simulink model "b_r309c_med"  (Simulink 6.2)
settings: Solver=ode45  StartTime=0.0  StopTime=1030.0  RelTol=1e-3
undefined symbols (not defined in the file): ant_bits, BEE2_usr, blockCountBits, blockRowBits, cmult_4bit_em
libraries: xbsIndex_r3 x2808, xps_library x97, casper_library x84
(part 1 of 20)
settings Model: LastModifiedBy=dsp
settings DebuggingCC: SolverPrmCheckMsg=warning

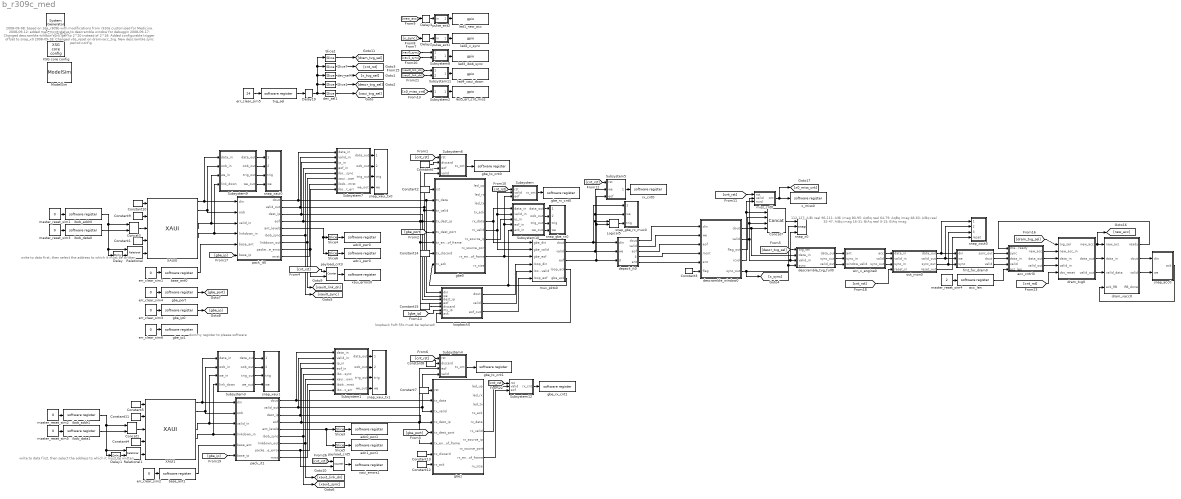
== system b_r309c_med ==
  note: 2008-09-08: based on 16a_r309b with modifications from r310a
      | customised for Medicina.
      |
      | 2008-09-12: added max_mcnt status to descramble window for debuggin
      |
      | 2008-09-17:
      | Changed descramble window sync gen to 2^20 instead of 2^18.
      | Added configurable trigger offset to snap_x0
      |
      | 2008-09-18:
      | Changed vbs_reset on dramvacc_tvg.
      | New descramble sync period config
  note: 112-127: AiBi real
      | 96-111: AiBi imag
      | 80-95: AqBq real
      | 64-79: AqBq imag
      | 48-63: AiBq real
      | 32-47: AiBq imag
      | 16-31: BiAq real
      | 0-15: BiAq imag
  note: write to data first,
      | then select the address
      | to which it must be written
  note: write to data first,
      | then select the address
      | to which it must be written
  note: loopback fwft fifo must be replaced!
  note: dummy register
      | to please software
  " System Generator" : xbsIndex_r3/ System Generator  Tag=genX  xilinxfamily=Virtex2P  part=xc2vp70  speed=-7  package=ff1704  synthesis_tool=XST  directory=./b_r309c_med/sysgen  testbench=off  simulink_period=1  sysclk_period=4.878  incr_netlist=off  trim_vbits=Everywhere in SubSystem  dbl_ovrd=According to Block Masks  core_generation=According to Block Masks  run_coregen=off  deprecated_control=off  eval_field=0
      settings: AttributesFormatString=System\nGenerator
  Concat1 : xbsIndex_r3/Concat  num_inputs=2  explicit_period=off  period=1  dbl_ovrd=off
  Concat3 : xbsIndex_r3/Concat  num_inputs=2  explicit_period=off  period=1  dbl_ovrd=off
  Concat7 : xbsIndex_r3/Concat  num_inputs=4  explicit_period=off  period=1  dbl_ovrd=off
  Constant1 : xbsIndex_r3/Constant  const=0  equ=P=C  arith_type=Unsigned  n_bits=64  bin_pt=0  opselect=C  inp2=PCIN>>17  opr=+  inp1=P  carry=CIN  iostate=0  explicit_period=on  period=1  dbl_ovrd=off
  Constant10 : xbsIndex_r3/Constant  const=1  equ=P=C  arith_type=Boolean  n_bits=1  bin_pt=0  opselect=C  inp2=PCIN>>17  opr=+  inp1=P  carry=CIN  iostate=0  explicit_period=on  period=1  dbl_ovrd=off
  Constant{2,6..7,9,11,14..15} (7 alike) : xbsIndex_r3/Constant  const=0  equ=P=C  arith_type=Boolean  n_bits=1  bin_pt=0  opselect=C  inp2=PCIN>>17  opr=+  inp1=P  carry=CIN  iostate=0  explicit_period=on  period=1  dbl_ovrd=off
  Constant12 : xbsIndex_r3/Constant  const=1  equ=P=C  arith_type=Boolean  n_bits=16  bin_pt=0  opselect=C  inp2=PCIN>>17  opr=+  inp1=P  carry=CIN  iostate=0  explicit_period=on  period=1  dbl_ovrd=off
  Constant13 : xbsIndex_r3/Constant  const=0  equ=P=C  arith_type=Boolean  n_bits=16  bin_pt=0  opselect=C  inp2=PCIN>>17  opr=+  inp1=P  carry=CIN  iostate=0  explicit_period=on  period=1  dbl_ovrd=off
  Constant3 : xbsIndex_r3/Constant  const=0  equ=P=C  arith_type=Unsigned  n_bits=1  bin_pt=0  opselect=C  inp2=PCIN>>17  opr=+  inp1=P  carry=CIN  iostate=0  explicit_period=on  period=1  dbl_ovrd=off
  Constant4 : xbsIndex_r3/Constant  const=0  equ=P=C  arith_type=Unsigned  n_bits=64  bin_pt=0  opselect=C  inp2=PCIN>>17  opr=+  inp1=P  carry=CIN  iostate=0  explicit_period=on  period=1  dbl_ovrd=off
  Constant5 : xbsIndex_r3/Constant  const=1  equ=P=C  arith_type=Boolean  n_bits=1  bin_pt=0  opselect=C  inp2=PCIN>>17  opr=+  inp1=P  carry=CIN  iostate=0  explicit_period=on  period=1  dbl_ovrd=off
  Constant8 : xbsIndex_r3/Constant  const=0  equ=P=C  arith_type=Boolean  n_bits=16  bin_pt=0  opselect=C  inp2=PCIN>>17  opr=+  inp1=P  carry=CIN  iostate=0  explicit_period=on  period=1  dbl_ovrd=off
  Delay{,1..3} (4 alike) : xbsIndex_r3/Delay  latency=1  reg_retiming=on  explicit_period=off  period=1  en=off  accept_only_valid=off  init_zero=on  dbl_ovrd=off  show_param=off
      settings: xl_area=[0, 0, 0, 0, 0, 0, 0]
  Delay19 : xbsIndex_r3/Delay  latency=2  reg_retiming=on  explicit_period=off  period=1  en=off  accept_only_valid=off  init_zero=on  dbl_ovrd=off  show_param=off
      settings: xl_area=[0, 0, 0, 0, 0, 0, 0]
  Logical5 : xbsIndex_r3/Logical  logical_function=AND  inputs=2  precision=Full  arith_type=Unsigned  n_bits=8  bin_pt=2  align_bp=on  latency=0  explicit_period=off  period=1  en=off  dbl_ovrd=off  show_param=off
      settings: xl_area=[0, 0, 0, 0, 0, 0, 0]
  ModelSim : xbsIndex_r3/ModelSim  dir=./modelsim  waveform=on  leave_open=on  skip_compile=off  custom_scripts=off  startup_timeout=40
  Relational : xbsIndex_r3/Relational  mode=a!=b  latency=0  explicit_period=off  period=1  en=off  dbl_ovrd=off  show_param=off
      settings: xl_area=[0, 0, 0, 0, 0, 0, 0]
  Relational1 : xbsIndex_r3/Relational  mode=a!=b  latency=0  explicit_period=off  period=1  en=off  dbl_ovrd=off  show_param=off
      settings: xl_area=[0, 0, 0, 0, 0, 0, 0]
  Slice1 : xbsIndex_r3/Slice  mode=Lower Bit Location + Width  nbits=2  bit1=0  base1=MSB of Input  bit0=1  base0=LSB of Input  boolean_output=off  explicit_period=off  period=1  dbl_ovrd=off
  Slice2 : xbsIndex_r3/Slice  mode=Lower Bit Location + Width  nbits=6  bit1=0  base1=MSB of Input  bit0=9  base0=LSB of Input  boolean_output=off  explicit_period=off  period=1  dbl_ovrd=off
  Slice3 : xbsIndex_r3/Slice  mode=Lower Bit Location + Width  nbits=32  bit1=0  base1=MSB of Input  bit0=32  base0=LSB of Input  boolean_output=off  explicit_period=off  period=1  dbl_ovrd=off
  Slice4 : xbsIndex_r3/Slice  mode=Lower Bit Location + Width  nbits=32  bit1=0  base1=MSB of Input  bit0=32  base0=LSB of Input  boolean_output=off  explicit_period=off  period=1  dbl_ovrd=off
  Slice5 : xbsIndex_r3/Slice  mode=Lower Bit Location + Width  nbits=32  bit1=0  base1=MSB of Input  bit0=0  base0=LSB of Input  boolean_output=off  explicit_period=off  period=1  dbl_ovrd=off
  Slice6 : xbsIndex_r3/Slice  mode=Lower Bit Location + Width  nbits=32  bit1=0  base1=MSB of Input  bit0=0  base0=LSB of Input  boolean_output=off  explicit_period=off  period=1  dbl_ovrd=off
  Slice7 : xbsIndex_r3/Slice  mode=Lower Bit Location + Width  nbits=1  bit1=0  base1=MSB of Input  bit0=8  base0=LSB of Input  boolean_output=on  explicit_period=off  period=1  dbl_ovrd=off
  Subsystem : Subsystem
  Subsystem1 : Subsystem
  Subsystem10 : Subsystem
  Subsystem11 : Subsystem
  Subsystem12 : Subsystem
  Subsystem2 : Subsystem
  Subsystem3 : Subsystem
  Subsystem4 : Subsystem
  Subsystem5 : Subsystem
  Subsystem6 : Subsystem
  Subsystem7 : Subsystem
  Subsystem8 : Subsystem
  Subsystem9 : Subsystem
  XAUI0 : xps_library/XAUI  Tag=xps:xaui  demux=1  port=BEE2_usr:0  show_param=off  pre_emph=3  swing=800
  XAUI1 : xps_library/XAUI  Tag=xps:xaui  demux=1  port=BEE2_usr:1  show_param=on  pre_emph=3  swing=800
  XSG core config : xps_library/XSG core config  Tag=xps:xsg  hw_sys=BEE2_usr  ibob_linux=off  clk_src=sys_clk2x  gpio_clk_io_group=iBOB:sma  gpio_clk_bit_index=0  clk_rate=205  sample_period=1  synthesis_tool=XST  mpc_type=powerpc405
  acc_cntrl0 : Subsystem
  acc_len : xps_library/software register  Tag=xps:sw_reg  io_dir=From Processor  arith_type=Unsigned  bitwidth=32  bin_pt=0  sample_period=1  gw_name=b_r309c_med_acc_len_user_data_out
  adc0_pwr0 : xps_library/software register  Tag=xps:sw_reg  io_dir=To Processor  arith_type=Unsigned  bitwidth=32  bin_pt=0  sample_period=1  gw_name=b_r309c_med_adc0_pwr0_user_data_in
  adc0_pwr1 : xps_library/software register  Tag=xps:sw_reg  io_dir=To Processor  arith_type=Unsigned  bitwidth=32  bin_pt=0  sample_period=1  gw_name=b_r309c_med_adc0_pwr1_user_data_in
  adc1_pwr0 : xps_library/software register  Tag=xps:sw_reg  io_dir=To Processor  arith_type=Unsigned  bitwidth=32  bin_pt=0  sample_period=1  gw_name=b_r309c_med_adc1_pwr0_user_data_in
  adc1_pwr1 : xps_library/software register  Tag=xps:sw_reg  io_dir=To Processor  arith_type=Unsigned  bitwidth=32  bin_pt=0  sample_period=1  gw_name=b_r309c_med_adc1_pwr1_user_data_in
  base_ant0 : xps_library/software register  Tag=xps:sw_reg  io_dir=From Processor  arith_type=Unsigned  bitwidth=32  bin_pt=0  sample_period=1  gw_name=b_r309c_med_base_ant0_user_data_out
  base_ant1 : xps_library/software register  Tag=xps:sw_reg  io_dir=From Processor  arith_type=Unsigned  bitwidth=32  bin_pt=0  sample_period=1  gw_name=b_r309c_med_base_ant1_user_data_out
  depack_it0 : Subsystem  mask{payload_len=32}
      mask prompts: payload_len "Payload Length"
      mask init:
      | payload_bits = ceil(log2(payload_len));
      | packet_len = payload_len + 1;
      | packet_bits = ceil(log2(packet_len));
  descramble_tvg_full0 : Subsystem  mask{ant_bits=4, x_int_bits=7, sync_period=20}
      mask prompts: ant_bits "Number of Antennas (2^?):"; x_int_bits "X Integration Length (2^?):"; sync_period "Sync Pulse Period (2^?):"
  descramble_window0 : Subsystem  mask{ant_bits=4, x_int_bits=7, window_bits=3, n_chans=2048, n_xeng=4}
      mask prompts: ant_bits "Maximum Number of Antennas (2^?):"; x_int_bits "X Engine Integration Length (2^?):"; window_bits "Number of Windows to Buffer (2^?):"; n_chans "Number of frequency channels in the system"; n_xeng "Number of Xengines in the system"
      mask init:
      | sync_clks=n_chans/n_xeng*(2^x_int_bits)*(2^ant_bits)
      | 
      | sync_bits=ceil(log2(sync_clks))
      | 
      | fmtstr = sprintf('Sync period: 2^%d', sync_bits);
      | set_param(gcb, 'AttributesFormatString', fmtstr);
      settings: AttributesFormatString=Sync period: 2^20
  dev_sel1 : xbsIndex_r3/Slice  mode=Lower Bit Location + Width  nbits=1  bit1=0  base1=MSB of Input  bit0=0  base0=LSB of Input  boolean_output=off  explicit_period=off  period=1  dbl_ovrd=off
  dev_sel4 : xbsIndex_r3/Slice  mode=Lower Bit Location + Width  nbits=2  bit1=0  base1=MSB of Input  bit0=3  base0=LSB of Input  boolean_output=off  explicit_period=off  period=1  dbl_ovrd=off
  dram_tvg0 : Subsystem  mask{len=(2048/4) * (16*17/2) * 4 * 2 / 4}
      mask prompts: len "Number of Vectors"
      mask init:
      | fmtstr = sprintf('Vector Length: %d', len);
      | set_param(gcb, 'AttributesFormatString', fmtstr);
      settings: AttributesFormatString=Vector Length: 139264
  dram_vacc0 : Subsystem  mask{acc_length=139264}
      mask prompts: acc_length "Vector length??(# cycles)"
      mask init:
      | valid_length = 36;
  err_clear_sim{1..4,6} (5 alike) : Constant  Value=0
  err_clear_sim5 : Constant  Value=24
  fmt_for_dram0 : Subsystem  mask{x_int_bits=7, x_n_bits=4}
      mask prompts: x_int_bits "X Engine integration length (2^?):"; x_n_bits "X Engine input bits"
  gbe0 : Subsystem  Tag=xps:tengbe  AncestorBlock=xps_library/ten_GbE  mask{port=BEE2_usr:2, mac_lite=on, show_param=off, pre_emph=3, swing=800}
      mask prompts: mac_lite "Use light-weight MAC: Warning --> it DOES NOT check any CRC on receive"; show_param "---------------------- Show Implementation Parameters -----------------------------------------------------------------------------------"; pre_emph "Pre-emphasis"; swing "Differential swing"
      mask init:
      | tengbe_mask;
      mask StyleString: popup(iBOB:0|iBOB:1|BEE2_ctrl:0|BEE2_ctrl:1|BEE2_usr:0|BEE2_usr:1|BEE2_usr:2|BEE2_usr:3|CORR:0),checkbox,checkbox,popup(0|1|2|3),popup(400|500|600|700|800)
      mask CallbackString:
      | ||myname=gcb;
      | if strcmp(get_param(myname, 'show_param'), 'on')
      |     set_param(myname, 'MaskVisibilities', {'on','on','on','on', 'on'});
      | else
      |     set_param(myname, 'MaskVisibilities', {'on','on','on','off','off'});
      | end||
  gbe1 : Subsystem  Tag=xps:tengbe  AncestorBlock=xps_library/ten_GbE  mask{port=BEE2_usr:3, mac_lite=on, show_param=off, pre_emph=3, swing=800}
      mask prompts: mac_lite "Use light-weight MAC: Warning --> it DOES NOT check any CRC on receive"; show_param "---------------------- Show Implementation Parameters -----------------------------------------------------------------------------------"; pre_emph "Pre-emphasis"; swing "Differential swing"
      mask init:
      | tengbe_mask;
      mask StyleString: popup(iBOB:0|iBOB:1|BEE2_ctrl:0|BEE2_ctrl:1|BEE2_usr:0|BEE2_usr:1|BEE2_usr:2|BEE2_usr:3|CORR:0),checkbox,checkbox,popup(0|1|2|3),popup(400|500|600|700|800)
      mask CallbackString:
      | ||myname=gcb;
      | if strcmp(get_param(myname, 'show_param'), 'on')
      |     set_param(myname, 'MaskVisibilities', {'on','on','on','on', 'on'});
      | else
      |     set_param(myname, 'MaskVisibilities', {'on','on','on','off','off'});
      | end||
  gbe_ip0 : xps_library/software register  Tag=xps:sw_reg  io_dir=From Processor  arith_type=Unsigned  bitwidth=32  bin_pt=0  sample_period=1  gw_name=b_r309c_med_gbe_ip0_user_data_out
  gbe_ip1 : xps_library/software register  Tag=xps:sw_reg  io_dir=From Processor  arith_type=Unsigned  bitwidth=32  bin_pt=0  sample_period=1  gw_name=b_r309c_med_gbe_ip1_user_data_out
  gbe_port : xps_library/software register  Tag=xps:sw_reg  io_dir=From Processor  arith_type=Unsigned  bitwidth=32  bin_pt=0  sample_period=1  gw_name=b_r309c_med_gbe_port_user_data_out
  gbe_rx_cnt0 : xps_library/software register  Tag=xps:sw_reg  io_dir=To Processor  arith_type=Unsigned  bitwidth=32  bin_pt=0  sample_period=1  gw_name=b_r309c_med_gbe_rx_cnt0_user_data_in
  gbe_rx_cnt1 : xps_library/software register  Tag=xps:sw_reg  io_dir=To Processor  arith_type=Unsigned  bitwidth=32  bin_pt=0  sample_period=1  gw_name=b_r309c_med_gbe_rx_cnt1_user_data_in
  gbe_tx_cnt0 : xps_library/software register  Tag=xps:sw_reg  io_dir=To Processor  arith_type=Unsigned  bitwidth=32  bin_pt=0  sample_period=1  gw_name=b_r309c_med_gbe_tx_cnt0_user_data_in
  gbe_tx_cnt1 : xps_library/software register  Tag=xps:sw_reg  io_dir=To Processor  arith_type=Unsigned  bitwidth=32  bin_pt=0  sample_period=1  gw_name=b_r309c_med_gbe_tx_cnt1_user_data_in
  ibob_addr0 : xps_library/software register  Tag=xps:sw_reg  io_dir=From Processor  arith_type=Unsigned  bitwidth=32  bin_pt=0  sample_period=1  gw_name=b_r309c_med_ibob_addr0_user_data_out
  ibob_addr1 : xps_library/software register  Tag=xps:sw_reg  io_dir=From Processor  arith_type=Unsigned  bitwidth=32  bin_pt=0  sample_period=1  gw_name=b_r309c_med_ibob_addr1_user_data_out
  ibob_data0 : xps_library/software register  Tag=xps:sw_reg  io_dir=From Processor  arith_type=Unsigned  bitwidth=32  bin_pt=0  sample_period=1  gw_name=b_r309c_med_ibob_data0_user_data_out
  ibob_data1 : xps_library/software register  Tag=xps:sw_reg  io_dir=From Processor  arith_type=Unsigned  bitwidth=32  bin_pt=0  sample_period=1  gw_name=b_r309c_med_ibob_data1_user_data_out
  led1_new_acc : xps_library/gpio  Tag=xps:gpio  io_group=BEE2_usr:led  io_dir=out  arith_type=Boolean  bitwidth=1  bin_pt=0  bit_index=0  sample_period=1  use_single_ended=off  use_ddr=off  reg_iob=off  reg_clk_phase=0  termination=None
  led2_x_sync : xps_library/gpio  Tag=xps:gpio  io_group=BEE2_usr:led  io_dir=out  arith_type=Boolean  bitwidth=1  bin_pt=0  bit_index=1  sample_period=1  use_single_ended=off  use_ddr=off  reg_iob=off  reg_clk_phase=0  termination=None
  led3_ibob_sync : xps_library/gpio  Tag=xps:gpio  io_group=BEE2_usr:led  io_dir=out  arith_type=Boolean  bitwidth=1  bin_pt=0  bit_index=2  sample_period=1  use_single_ended=off  use_ddr=off  reg_iob=off  reg_clk_phase=0  termination=None
  led4_xaui_down : xps_library/gpio  Tag=xps:gpio  io_group=BEE2_usr:led  io_dir=out  arith_type=Boolean  bitwidth=1  bin_pt=0  bit_index=3  sample_period=1  use_single_ended=off  use_ddr=off  reg_iob=off  reg_clk_phase=0  termination=None
  led5_err_cnt_miss : xps_library/gpio  Tag=xps:gpio  io_group=BEE2_usr:led  io_dir=out  arith_type=Boolean  bitwidth=1  bin_pt=0  bit_index=4  sample_period=1  use_single_ended=off  use_ddr=off  reg_iob=off  reg_clk_phase=0  termination=None
  loopback0 : Subsystem  mask{depth_bits=8}
      mask prompts: depth_bits "Buffer Size (2^?):"
      mask help: A loopback is a buffer for holding packets which are to be transmitted to one's self. Most switches drop any packets which have a destination IP address equal to the address of the transmitter. Thus, a seperate buffer is needed to collect these packets for readback.
  master_reset_sim{1..3,5} (4 alike) : Constant  Value=0
  master_reset_sim4 : Constant  Value=2
  miss_cnt0 : Subsystem
  mux_pkts0 : Subsystem
  out_mon0 : Subsystem  mask{n_ants=16, n_chans=2048, n_xeng=4}
      mask prompts: n_ants "Number of Antennas"; n_chans "Number of Frequency Channels in the system"; n_xeng "Number of X engines"
  pack_it0 : Subsystem  mask{payload_len=32, ant_bits=4, xeng_bits=2, skip_xeng_bits=0, skip_ant_bits=1}
      mask prompts: payload_len "Payload Length (in 64 bit words)"; ant_bits "Number of Antennas (2^?)"; xeng_bits "Number of X engines (2^?)"; skip_xeng_bits "X engines per IP address (2^?)"; skip_ant_bits "Antennas per XAUI link (2^?)"
      mask help: Packetizes data coming in over a XAUI interface. A packet consists of a 64 bit header (48 bits of "mcnt" and 16 bits of antenna), followed by 64 x "payload" bits of payload. "Mcnt" (master count) is a counter which keeps track of how many packets have been transmitted since the last "mrst".
      mask init:
      | packet_len = payload_len + 1;
      | packet_bits = ceil(log2(packet_len));
      | payload_bits = ceil(log2(payload_len));
  pack_it1 : Subsystem  mask{payload_len=32, ant_bits=4, xeng_bits=2, skip_xeng_bits=0, skip_ant_bits=1}
      mask prompts: payload_len "Payload Length (in 64 bit words)"; ant_bits "Number of Antennas (2^?)"; xeng_bits "Number of X engines (2^?)"; skip_xeng_bits "X engines per IP address (2^?)"; skip_ant_bits "Antennas per XAUI link (2^?)"
      mask help: Packetizes data coming in over a XAUI interface. A packet consists of a 64 bit header (48 bits of "mcnt" and 16 bits of antenna), followed by 64 x "payload" bits of payload. "Mcnt" (master count) is a counter which keeps track of how many packets have been transmitted since the last "mrst".
      mask init:
      | packet_len = payload_len + 1;
      | packet_bits = ceil(log2(packet_len));
      | payload_bits = ceil(log2(payload_len));
  payload_cnt3 : xbsIndex_r3/Counter  cnt_type=Free Running  n_bits=32  bin_pt=0  arith_type=Unsigned  start_count=0  cnt_to=0  cnt_by_val=1  operation=Up  explicit_period=off  period=1  load_pin=off  rst=on  en=on  dbl_ovrd=off  show_param=off  use_rpm=on  gen_core=off
      settings: xl_area=[0, 0, 0, 0, 0, 0, 0]
  payload_cnt5 : xbsIndex_r3/Counter  cnt_type=Free Running  n_bits=32  bin_pt=0  arith_type=Unsigned  start_count=0  cnt_to=0  cnt_by_val=1  operation=Up  explicit_period=off  period=1  load_pin=off  rst=on  en=on  dbl_ovrd=off  show_param=off  use_rpm=on  gen_core=off
      settings: xl_area=[0, 0, 0, 0, 0, 0, 0]
  pulse_ext1 : Subsystem  mask{pulse_len=2^23}
      mask prompts: pulse_len "Length of Pulse"
      mask init:
      | bits = ceil(log2(pulse_len));
  pulse_ext2 : Subsystem  mask{pulse_len=2^23}
      mask prompts: pulse_len "Length of Pulse"
      mask init:
      | bits = ceil(log2(pulse_len));
  rx_cnt0 : xps_library/software register  Tag=xps:sw_reg  io_dir=To Processor  arith_type=Unsigned  bitwidth=32  bin_pt=0  sample_period=1  gw_name=b_r309c_med_rx_cnt0_user_data_in
  snap_acc0 : Subsystem
  snap_gbe_rx0 : Subsystem  AncestorBlock=casper_library/Scopes/snap64  mask(snap64){nsamples=11}
      mask prompts: nsamples "No. of samples(2^?)"
      mask help:
      | The <i>snap</i> block provides a packaged solution to capturing data from
      | the FPGA fabric and making it accessible from the CPU.  The block comes in
      | 2 flavors: <i>snap</i> (which captures to a 32 bit wide Shared BRAM), and
      | <i>snap64</i> (which captures to 2x32 bit wide Shared BRAMs to effect a
      | 64 bit capture).
      mask Help: eval('xlWeb([getenv(''MLIB_ROOT''), ''\casper_library\doc\snap_usage.html''])')
  snap_gbe_rx_mux0 : Subsystem  AncestorBlock=casper_library/Scopes/snap64  mask(snap64){nsamples=12}
      mask prompts: nsamples "No. of samples(2^?)"
      mask help:
      | The <i>snap</i> block provides a packaged solution to capturing data from
      | the FPGA fabric and making it accessible from the CPU.  The block comes in
      | 2 flavors: <i>snap</i> (which captures to a 32 bit wide Shared BRAM), and
      | <i>snap64</i> (which captures to 2x32 bit wide Shared BRAMs to effect a
      | 64 bit capture).
      mask Help: eval('xlWeb([getenv(''MLIB_ROOT''), ''\casper_library\doc\snap_usage.html''])')
  snap_x0 : casper_library/Scopes/snap  nsamples=12
  snap_xaui0 : Subsystem  AncestorBlock=casper_library/Scopes/snap64  mask(snap64){nsamples=12}
      mask prompts: nsamples "No. of samples(2^?)"
      mask help:
      | The <i>snap</i> block provides a packaged solution to capturing data from
      | the FPGA fabric and making it accessible from the CPU.  The block comes in
      | 2 flavors: <i>snap</i> (which captures to a 32 bit wide Shared BRAM), and
      | <i>snap64</i> (which captures to 2x32 bit wide Shared BRAMs to effect a
      | 64 bit capture).
      mask Help: eval('xlWeb([getenv(''MLIB_ROOT''), ''\casper_library\doc\snap_usage.html''])')
  snap_xaui1 : Subsystem  AncestorBlock=casper_library/Scopes/snap64  mask(snap64){nsamples=12}
      mask prompts: nsamples "No. of samples(2^?)"
      mask help:
      | The <i>snap</i> block provides a packaged solution to capturing data from
      | the FPGA fabric and making it accessible from the CPU.  The block comes in
      | 2 flavors: <i>snap</i> (which captures to a 32 bit wide Shared BRAM), and
      | <i>snap64</i> (which captures to 2x32 bit wide Shared BRAMs to effect a
      | 64 bit capture).
      mask Help: eval('xlWeb([getenv(''MLIB_ROOT''), ''\casper_library\doc\snap_usage.html''])')
  snap_xaui_tx0 : Subsystem  AncestorBlock=casper_library/Scopes/snap64  mask(snap64){nsamples=11}
      mask prompts: nsamples "No. of samples(2^?)"
      mask help:
      | The <i>snap</i> block provides a packaged solution to capturing data from
      | the FPGA fabric and making it accessible from the CPU.  The block comes in
      | 2 flavors: <i>snap</i> (which captures to a 32 bit wide Shared BRAM), and
      | <i>snap64</i> (which captures to 2x32 bit wide Shared BRAMs to effect a
      | 64 bit capture).
      mask Help: eval('xlWeb([getenv(''MLIB_ROOT''), ''\casper_library\doc\snap_usage.html''])')
  snap_xaui_tx1 : Subsystem  AncestorBlock=casper_library/Scopes/snap64  mask(snap64){nsamples=11}
      mask prompts: nsamples "No. of samples(2^?)"
      mask help:
      | The <i>snap</i> block provides a packaged solution to capturing data from
      | the FPGA fabric and making it accessible from the CPU.  The block comes in
      | 2 flavors: <i>snap</i> (which captures to a 32 bit wide Shared BRAM), and
      | <i>snap64</i> (which captures to 2x32 bit wide Shared BRAMs to effect a
      | 64 bit capture).
      mask Help: eval('xlWeb([getenv(''MLIB_ROOT''), ''\casper_library\doc\snap_usage.html''])')
  snap_xout0 : Subsystem
  tvg_sel : xps_library/software register  Tag=xps:sw_reg  io_dir=From Processor  arith_type=Unsigned  bitwidth=32  bin_pt=0  sample_period=1  gw_name=b_r309c_med_tvg_sel_user_data_out
  win_x_engine0 : Subsystem  AncestorBlock=casper_library/Correlator/win_x_engine  mask(win_x_engine){n_ants=16, n_bits=4, acc_len=128, add_latency=1, mult_latency=1, bram_latency=1, use_ded_mult=1, use_bram_delay=1}
      mask prompts: n_ants "Number of antennas"; n_bits "Bit-width of samples in"; acc_len "Accumulation length"; add_latency "Adder latency"; mult_latency "Multiplier latency"; bram_latency "BRAM latency"; use_ded_mult "Implementation: Multiplier type (0=slices 1=embedded 2=bram)"; use_bram_delay "Implementation: Delay type (0=SLR, 1=BRAM)"
      mask help: CASPER X engine with added internal valid data masking functionality. Based on Aaron Parsons' design.
      mask init:
      | bit_growth = ceil(log2(acc_len));
      | ant_bits = ceil(log2(n_ants));
      | n_bits_out = (2*n_bits + 1 + bit_growth);
      | 
      | win_x_engine_init(gcb, ...
      |     'n_ants', n_ants, ...
      |     'n_bits', n_bits, ...
      |     'acc_len', acc_len, ...
      |     'add_latency', add_latency, ...
      |     'mult_latency', mult_latency, ...
      |     'bram_latency', bram_latency, ...
      |     'use_ded_mult', use_ded_mult, ...
      |     'use_bram_delay', use_bram_delay);
      settings: AttributesFormatString=n_ant=16, bits=4, mult=1, bram=1
      mask Help: eval('xlWeb([getenv(''MLIB_ROOT''), ''\doc\html\win_x_engine\win_x_engine.html''])')
  x_miss0 : xps_library/software register  Tag=xps:sw_reg  io_dir=To Processor  arith_type=Unsigned  bitwidth=32  bin_pt=0  sample_period=1  gw_name=b_r309c_med_x_miss0_user_data_in
  xaui_errors0 : xps_library/software register  Tag=xps:sw_reg  io_dir=To Processor  arith_type=Unsigned  bitwidth=32  bin_pt=0  sample_period=1  gw_name=b_r309c_med_xaui_errors0_user_data_in
  xaui_errors1 : xps_library/software register  Tag=xps:sw_reg  io_dir=To Processor  arith_type=Unsigned  bitwidth=32  bin_pt=0  sample_period=1  gw_name=b_r309c_med_xaui_errors1_user_data_in
  wires:
  err_clear_sim4/1 -> gbe_port/1
  err_clear_sim1/1 -> base_ant0/1
  Constant2/1 -> gbe0/1(rst)
  gbe0/9(rx_end_of_frame) -> mux_pkts0/3(gbe_eof), Subsystem10/4(eof_in), Subsystem/3(eof)
  err_clear_sim3/1 -> gbe_ip0/1
  mux_pkts0/1(dout) -> depack_it0/1(din), snap_gbe_rx_mux0/1(data_in)
  mux_pkts0/2(valid) -> depack_it0/2(we), Subsystem5/2(we), snap_gbe_rx_mux0/2(we), Logical5/1
  mux_pkts0/3(eof) -> depack_it0/3(eof_in), Logical5/2, Subsystem5/3(eof)
  loopback0/1(dout) -> mux_pkts0/4(loop_din)
  loopback0/2(valid) -> mux_pkts0/5(loop_valid)
  loopback0/3(eof_out) -> mux_pkts0/6(loop_eof)
  mux_pkts0/4(loop_ack) -> loopback0/7(ack)
  err_clear_sim5/1 -> tvg_sel/1
  tvg_sel/1 -> Delay19/1
  Delay19/1 -> dev_sel1/1, Slice1/1, dev_sel4/1, Slice2/1, Slice7/1
  dev_sel1/1 -> [xaui_tvg_sel]
  Slice1/1 -> [descr_tvg_sel]
  dev_sel4/1 -> [x_tvg_sel]
  Slice7/1 -> [cnt_rst]
  mux_pkts0/5(gbe_ack) -> gbe0/8(rx_ack), Subsystem10/5(ack_in)
  Subsystem8/1(Out1) -> led3_ibob_sync/1
  pulse_ext1/1(out) -> led2_x_sync/1
  Delay2/1 -> pulse_ext1/1(in)
  [x_sync] -> Delay2/1
  [x0_miss_cnt] -> Subsystem2/1(In1)
  Subsystem2/1(Out1) -> led5_err_cnt_miss/1
  Slice2/1 -> [dram_tvg_sel]
  pulse_ext2/1(out) -> led1_new_acc/1
  Delay3/1 -> pulse_ext2/1(in)
  [new_acc] -> Delay3/1
  Slice4/1 -> adc0_pwr0/1
  Slice6/1 -> adc1_pwr0/1
  [cnt_rst] -> payload_cnt3/1
  payload_cnt3/1 -> xaui_errors0/1
  pack_it0/1(dout) -> gbe0/2(tx_data), loopback0/1(din), Subsystem7/1(data_in)
  pack_it0/2(valid_out) -> gbe0/3(tx_valid), loopback0/2(we), Subsystem6/4(valid), Subsystem7/2(valid_in)
  pack_it0/3(dest_ip) -> gbe0/4(tx_dest_ip), loopback0/3(dest_ip), Subsystem7/3(ip_in)
  pack_it0/4(eof) -> gbe0/6(tx_end_of_frame), loopback0/4(eof), Subsystem6/3(eof), Subsystem7/4(eof_in)
  XAUI0/1 -> pack_it0/1(din), Subsystem9/1(data_in)
  XAUI0/4 -> pack_it0/3(valid_in), Subsystem9/3(we_in)
  XAUI0/5 -> pack_it0/4(linkdown_in), Subsystem9/4(link_down)
  base_ant0/1 -> pack_it0/5(base_ant)
  pack_it0/6(ibob_sync) -> Subsystem7/5(ibob_sync), [xaui0_sync]
  pack_it0/7(linkdown_out) -> Subsystem7/6(xaui_down), [xaui0_link_dn]
  pack_it0/5(ant_levels) -> Slice4/1, Slice6/1
  master_reset_sim3/1 -> ibob_data0/1
  master_reset_sim1/1 -> ibob_addr0/1
  ibob_data0/1 -> Concat3/2
  ibob_addr0/1 -> Concat3/1, Relational/1, Delay/1
  Constant10/1 -> XAUI0/1
  Constant9/1 -> XAUI0/2
  Concat3/1 -> XAUI0/3
  Constant1/1 -> XAUI0/4
  XAUI0/2 -> pack_it0/2(oob), Subsystem9/2(oob_in)
  pack_it0/9(mrst) -> Subsystem7/7(ibob_mrst)
  pack_it0/8(packet_size_error) -> Subsystem7/8(ibob_pkt_err), payload_cnt3/2
  depack_it0/2(valid) -> descramble_window0/2(we)
  depack_it0/4(mcnt) -> descramble_window0/4(mcnt)
  depack_it0/1(dout) -> descramble_window0/1(din)
  depack_it0/3(eof) -> descramble_window0/3(eof)
  depack_it0/5(ant) -> descramble_window0/5(ant)
  Constant3/1 -> descramble_window0/6(flag)
  descramble_window0/1(dout) -> Concat7/4, descramble_tvg_full0/2(data_in)
  descramble_window0/3(flag_out) -> Concat7/2
  descramble_window0/4(rcvd) -> Concat7/1, miss_cnt0/3(rcvd)
  descramble_window0/5(sync_out) -> snap_x0/2, descramble_tvg_full0/4(sync), [x_sync]
  descramble_window0/2(valid) -> Concat7/3, miss_cnt0/2(valid), snap_x0/3, descramble_tvg_full0/3(valid_in)
  miss_cnt0/1(cnt) -> x_miss0/1, [x0_miss_cnt]
  [cnt_rst] -> miss_cnt0/1(rst)
  [descr_tvg_sel] -> descramble_tvg_full0/1(tvg_sel)
  Concat7/1 -> snap_x0/1
  [cnt_rst] -> out_mon0/4(reset_in)
  out_mon0/3(sync_out) -> fmt_for_dram0/3(sync), snap_xout0/3(trigger)
  out_mon0/4(reset_out) -> snap_xout0/4(reset)
  out_mon0/2(valid_out) -> fmt_for_dram0/2(we), snap_xout0/2(valid_in)
  out_mon0/1(data_out) -> fmt_for_dram0/1(din), snap_xout0/1(data_in)
  acc_len/1 -> acc_cntrl0/5(acc_len)
  master_reset_sim4/1 -> acc_len/1
  dram_vacc0/2(dout) -> snap_acc0/1(din)
  dram_vacc0/3(valid) -> snap_acc0/2(we)
  snap_acc0/1(ack) -> dram_vacc0/4(ack_RB)
  dram_tvg0/1(new_acc) -> [new_acc], dram_vacc0/1(new_acc)
  dram_tvg0/2(data_out) -> dram_vacc0/2(data_in)
  dram_tvg0/3(valid_out) -> dram_vacc0/3(valid_data)
  [dram_tvg_sel] -> dram_tvg0/1(tvg_sel)
  fmt_for_dram0/1(sync_out) -> acc_cntrl0/2(sync)
  fmt_for_dram0/2(dout) -> acc_cntrl0/3(data_in)
  fmt_for_dram0/3(valid) -> acc_cntrl0/4("valid ")
  dram_vacc0/1(ready) -> acc_cntrl0/1(dram_ready)
  acc_cntrl0/1(new_acc) -> dram_tvg0/2(new_acc_in)
  acc_cntrl0/2(data_out) -> dram_tvg0/3(data_in)
  descramble_tvg_full0/1(data_out) -> win_x_engine0/1(ant)
  descramble_tvg_full0/2(sync_out) -> win_x_engine0/2(sync_in)
  descramble_tvg_full0/3(valid_out) -> win_x_engine0/3(window_valid)
  win_x_engine0/1(acc) -> out_mon0/1(data_in)
  win_x_engine0/2(valid) -> out_mon0/2(valid_in)
  win_x_engine0/3(sync_out) -> out_mon0/3(sync_in)
  Relational/1 -> XAUI0/5
  Delay/1 -> Relational/2
  acc_cntrl0/3(valid_out) -> dram_tvg0/4(valid_in)
  Subsystem7/1(data_out) -> snap_xaui_tx0/1(data_in)
  Subsystem7/2(oob_out) -> snap_xaui_tx0/2(oob_in)
  Subsystem7/3(trig_out) -> snap_xaui_tx0/3(trig)
  Subsystem7/4(we_out) -> snap_xaui_tx0/4(we)
  Subsystem9/1(data_out) -> snap_xaui0/1(data_in)
  Subsystem9/2(oob_out) -> snap_xaui0/2(oob_in)
  Subsystem9/3(trig_out) -> snap_xaui0/3(trig)
  Subsystem9/4(we_out) -> snap_xaui0/4(we)
  err_clear_sim2/1 -> base_ant1/1
  Constant7/1 -> gbe1/1(rst)
  Slice3/1 -> adc0_pwr1/1
  Slice5/1 -> adc1_pwr1/1
  [cnt_rst] -> payload_cnt5/1
  payload_cnt5/1 -> xaui_errors1/1
  pack_it1/1(dout) -> Subsystem1/1(data_in), gbe1/2(tx_data)
  pack_it1/2(valid_out) -> gbe1/3(tx_valid), Subsystem4/4(valid), Subsystem1/2(valid_in)
  pack_it1/3(dest_ip) -> Subsystem1/3(ip_in), gbe1/4(tx_dest_ip)
  pack_it1/4(eof) -> gbe1/6(tx_end_of_frame), Subsystem4/3(eof), Subsystem1/4(eof_in)
  XAUI1/1 -> pack_it1/1(din), Subsystem3/1(data_in)
  XAUI1/4 -> pack_it1/3(valid_in), Subsystem3/3(we_in)
  XAUI1/5 -> pack_it1/4(linkdown_in), Subsystem3/4(link_down)
  base_ant1/1 -> pack_it1/5(base_ant)
  pack_it1/5(ant_levels) -> Slice3/1, Slice5/1
  master_reset_sim5/1 -> ibob_data1/1
  master_reset_sim2/1 -> ibob_addr1/1
  ibob_data1/1 -> Concat1/2
  ibob_addr1/1 -> Concat1/1, Relational1/1, Delay1/1
  Constant5/1 -> XAUI1/1
  Constant11/1 -> XAUI1/2
  Concat1/1 -> XAUI1/3
  Constant4/1 -> XAUI1/4
  XAUI1/2 -> pack_it1/2(oob), Subsystem3/2(oob_in)
  Relational1/1 -> XAUI1/5
  Delay1/1 -> Relational1/2
  Subsystem1/1(data_out) -> snap_xaui_tx1/1(data_in)
  Subsystem1/2(oob_out) -> snap_xaui_tx1/2(oob_in)
  Subsystem1/3(trig_out) -> snap_xaui_tx1/3(trig)
  Subsystem1/4(we_out) -> snap_xaui_tx1/4(we)
  Subsystem3/1(data_out) -> snap_xaui1/1(data_in)
  Subsystem3/2(oob_out) -> snap_xaui1/2(oob_in)
  Subsystem3/3(trig_out) -> snap_xaui1/3(trig)
  Subsystem3/4(we_out) -> snap_xaui1/4(we)
  Subsystem4/1(tx_cnt) -> gbe_tx_cnt1/1
  [cnt_rst] -> Subsystem4/1(rst)
  Constant12/1 -> gbe1/8(rx_ack)
  pack_it1/8(packet_size_error) -> payload_cnt5/2, Subsystem1/8(ibob_pkt_err)
  pack_it1/6(ibob_sync) -> Subsystem1/5(ibob_sync), [xaui1_sync]
  pack_it1/7(linkdown_out) -> Subsystem1/6(xaui_down), [xaui1_link_dn]
  pack_it1/9(mrst) -> Subsystem1/7(ibob_mrst)
  Subsystem/1(rx_cnt) -> gbe_rx_cnt0/1
  [cnt_rst] -> Subsystem/1(rst)
  Subsystem5/1(rx_cnt) -> rx_cnt0/1
  [cnt_rst] -> Subsystem5/1(rst)
  Logical5/1 -> snap_gbe_rx_mux0/3(trig)
  Subsystem10/1(data_out) -> snap_gbe_rx0/1(data_in)
  Subsystem10/2(oob_out) -> snap_gbe_rx0/2(oob_in)
  Subsystem10/3(trig_out) -> snap_gbe_rx0/3(trig)
  Subsystem10/4(we_out) -> snap_gbe_rx0/4(we)
  Subsystem6/1(tx_cnt) -> gbe_tx_cnt0/1
  [cnt_rst] -> Subsystem6/1(rst)
  gbe0/5(rx_data) -> Subsystem10/1(data_in), mux_pkts0/1(gbe_din)
  gbe0/6(rx_valid) -> Subsystem10/2(valid_in), Subsystem/2(valid), mux_pkts0/2(gbe_valid)
  gbe0/7(rx_source_ip) -> Subsystem10/3(ip_in)
  gbe_port/1 -> [gbe_port]
  [gbe_port] -> gbe0/5(tx_dest_port)
  [gbe_port] -> gbe1/5(tx_dest_port)
  Constant13/1 -> gbe1/7(tx_discard)
  Constant8/1 -> Subsystem4/2(discard)
  Constant6/1 -> Subsystem6/2(discard)
  Constant14/1 -> gbe0/7(tx_discard)
  Constant15/1 -> loopback0/5(discard)
  gbe_ip0/1 -> [gbe_ip]
  [gbe_ip] -> loopback0/6(my_ip)
  [gbe_ip] -> pack_it0/6(base_ip)
  [gbe_ip] -> pack_it1/6(base_ip)
  [xaui0_sync] -> Subsystem8/1(In1)
  [xaui1_sync] -> Subsystem8/2(In2)
  Subsystem11/1(Out1) -> led4_xaui_down/1
  [xaui0_link_dn] -> Subsystem11/1(In1)
  [xaui1_link_dn] -> Subsystem11/2(In2)
  err_clear_sim6/1 -> gbe_ip1/1
  Subsystem12/1(rx_cnt) -> gbe_rx_cnt1/1
  [cnt_rst] -> Subsystem12/1(rst)
  gbe1/6(rx_valid) -> Subsystem12/2(valid)
  gbe1/9(rx_end_of_frame) -> Subsystem12/3(eof)
  [cnt_rst] -> dram_tvg0/5(vbs_reset)

== system b_r309c_med/Subsystem ==
  rst : Inport  Port=1  LatchInput=off
  valid : Inport  Port=2  LatchInput=off
  eof : Inport  Port=3  LatchInput=off
  Logical4 : xbsIndex_r3/Logical  logical_function=AND  inputs=2  precision=Full  arith_type=Unsigned  n_bits=8  bin_pt=2  align_bp=on  latency=0  explicit_period=on  period=1  en=off  dbl_ovrd=off  show_param=off
      settings: xl_area=[0, 0, 0, 0, 0, 0, 0]
  payload_cnt2 : xbsIndex_r3/Counter  cnt_type=Free Running  n_bits=32  bin_pt=0  arith_type=Unsigned  start_count=0  cnt_to=0  cnt_by_val=1  operation=Up  explicit_period=on  period=1  load_pin=off  rst=on  en=on  dbl_ovrd=off  show_param=off  use_rpm=on  gen_core=off
      settings: xl_area=[0, 0, 0, 0, 0, 0, 0]
  posedge1 : casper_library/Misc/posedge  Tag=Rising Edge Detector
  rx_cnt : Outport
  wires:
  Logical4/1 -> posedge1/1
  posedge1/1 -> payload_cnt2/2
  valid/1 -> Logical4/1
  eof/1 -> Logical4/2
  rst/1 -> payload_cnt2/1
  payload_cnt2/1 -> rx_cnt/1

== system b_r309c_med/Subsystem1 ==
  note: Trigger the snap block
      | one clock cycle before
      | first valid data to ensure
      | its capture.
  data_in : Inport  Port=1  LatchInput=off
  valid_in : Inport  Port=2  LatchInput=off
  ip_in : Inport  Port=3  LatchInput=off
  eof_in : Inport  Port=4  LatchInput=off
  ibob_sync : Inport  Port=5  LatchInput=off
  xaui_down : Inport  Port=6  LatchInput=off
  ibob_mrst : Inport  Port=7  LatchInput=off
  ibob_pkt_err : Inport  Port=8  LatchInput=off
  Concat1 : xbsIndex_r3/Concat  num_inputs=6  explicit_period=off  period=1  dbl_ovrd=off
  Delay{1..4} (4 alike) : xbsIndex_r3/Delay  latency=2  reg_retiming=on  explicit_period=off  period=1  en=off  accept_only_valid=off  init_zero=on  dbl_ovrd=off  show_param=off
      settings: xl_area=[0, 0, 0, 0, 0, 0, 0]
  Logical4 : xbsIndex_r3/Logical  logical_function=AND  inputs=2  precision=Full  arith_type=Unsigned  n_bits=8  bin_pt=2  align_bp=on  latency=0  explicit_period=on  period=1  en=off  dbl_ovrd=off  show_param=off
      settings: xl_area=[0, 0, 0, 0, 0, 0, 0]
  Slice11 : xbsIndex_r3/Slice  mode=Lower Bit Location + Width  nbits=24  bit1=0  base1=MSB of Input  bit0=0  base0=LSB of Input  boolean_output=on  explicit_period=off  period=1  dbl_ovrd=off
  data_out : Outport
  oob_out : Outport  Port=2
  trig_out : Outport  Port=3
  we_out : Outport  Port=4
  wires:
  Slice11/1 -> Concat1/1
  Concat1/1 -> Delay4/1
  data_in/1 -> Delay1/1
  ip_in/1 -> Slice11/1
  Delay1/1 -> data_out/1
  Delay4/1 -> oob_out/1
  Logical4/1 -> Delay3/1
  valid_in/1 -> Logical4/2, Delay2/1
  eof_in/1 -> Concat1/2
  ibob_sync/1 -> Concat1/3, Logical4/1
  xaui_down/1 -> Concat1/4
  ibob_mrst/1 -> Concat1/5
  ibob_pkt_err/1 -> Concat1/6
  Delay2/1 -> we_out/1
  Delay3/1 -> trig_out/1

== system b_r309c_med/Subsystem10 ==
  note: Trigger the snap block
      | one clock cycle before
      | first valid data to ensure
      | its capture.
  data_in : Inport  Port=1  LatchInput=off
  valid_in : Inport  Port=2  LatchInput=off
  ip_in : Inport  Port=3  LatchInput=off
  eof_in : Inport  Port=4  LatchInput=off
  ack_in : Inport  Port=5  LatchInput=off
  Concat1 : xbsIndex_r3/Concat  num_inputs=2  explicit_period=off  period=1  dbl_ovrd=off
  Delay{1..4} (4 alike) : xbsIndex_r3/Delay  latency=2  reg_retiming=on  explicit_period=off  period=1  en=off  accept_only_valid=off  init_zero=on  dbl_ovrd=off  show_param=off
      settings: xl_area=[0, 0, 0, 0, 0, 0, 0]
  Logical1 : xbsIndex_r3/Logical  logical_function=AND  inputs=2  precision=Full  arith_type=Unsigned  n_bits=8  bin_pt=2  align_bp=on  latency=0  explicit_period=on  period=1  en=off  dbl_ovrd=off  show_param=off
      settings: xl_area=[0, 0, 0, 0, 0, 0, 0]
  Logical4 : xbsIndex_r3/Logical  logical_function=AND  inputs=2  precision=Full  arith_type=Unsigned  n_bits=8  bin_pt=2  align_bp=on  latency=0  explicit_period=on  period=1  en=off  dbl_ovrd=off  show_param=off
      settings: xl_area=[0, 0, 0, 0, 0, 0, 0]
  Slice11 : xbsIndex_r3/Slice  mode=Lower Bit Location + Width  nbits=32-1  bit1=0  base1=MSB of Input  bit0=0  base0=LSB of Input  boolean_output=on  explicit_period=off  period=1  dbl_ovrd=off
  data_out : Outport
  oob_out : Outport  Port=2
  trig_out : Outport  Port=3
  we_out : Outport  Port=4
  wires:
  Slice11/1 -> Concat1/1
  Concat1/1 -> Delay4/1
  data_in/1 -> Delay1/1
  ip_in/1 -> Slice11/1
  Delay1/1 -> data_out/1
  Delay4/1 -> oob_out/1
  Logical4/1 -> Delay2/1
  valid_in/1 -> Logical1/1
  eof_in/1 -> Concat1/2, Logical4/1
  ack_in/1 -> Logical1/2
  Logical1/1 -> Logical4/2, Delay3/1
  Delay2/1 -> trig_out/1
  Delay3/1 -> we_out/1

== system b_r309c_med/Subsystem11 ==
  In1 : Inport  Port=1  LatchInput=off
  In2 : Inport  Port=2  LatchInput=off
  Delay1 : xbsIndex_r3/Delay  latency=1  reg_retiming=on  explicit_period=off  period=1  en=off  accept_only_valid=off  init_zero=on  dbl_ovrd=off  show_param=off
      settings: xl_area=[0, 0, 0, 0, 0, 0, 0]
  Delay8 : xbsIndex_r3/Delay  latency=1  reg_retiming=on  explicit_period=off  period=1  en=off  accept_only_valid=off  init_zero=on  dbl_ovrd=off  show_param=off
      settings: xl_area=[0, 0, 0, 0, 0, 0, 0]
  Logical : xbsIndex_r3/Logical  logical_function=OR  inputs=2  precision=Full  arith_type=Unsigned  n_bits=8  bin_pt=2  align_bp=on  latency=0  explicit_period=off  period=1  en=off  dbl_ovrd=off  show_param=off
      settings: xl_area=[0, 0, 0, 0, 0, 0, 0]
  pulse_ext : Subsystem  mask{pulse_len=2^23}
      mask prompts: pulse_len "Length of Pulse"
      mask init:
      | bits = ceil(log2(pulse_len));
  Out1 : Outport
  wires:
  Delay1/1 -> Logical/2
  Delay8/1 -> Logical/1
  In2/1 -> Delay1/1
  Logical/1 -> pulse_ext/1(in)
  pulse_ext/1(out) -> Out1/1
  In1/1 -> Delay8/1

== system b_r309c_med/Subsystem12 ==
  rst : Inport  Port=1  LatchInput=off
  valid : Inport  Port=2  LatchInput=off
  eof : Inport  Port=3  LatchInput=off
  Logical4 : xbsIndex_r3/Logical  logical_function=AND  inputs=2  precision=Full  arith_type=Unsigned  n_bits=8  bin_pt=2  align_bp=on  latency=0  explicit_period=on  period=1  en=off  dbl_ovrd=off  show_param=off
      settings: xl_area=[0, 0, 0, 0, 0, 0, 0]
  payload_cnt2 : xbsIndex_r3/Counter  cnt_type=Free Running  n_bits=32  bin_pt=0  arith_type=Unsigned  start_count=0  cnt_to=0  cnt_by_val=1  operation=Up  explicit_period=on  period=1  load_pin=off  rst=on  en=on  dbl_ovrd=off  show_param=off  use_rpm=on  gen_core=off
      settings: xl_area=[0, 0, 0, 0, 0, 0, 0]
  posedge1 : casper_library/Misc/posedge  Tag=Rising Edge Detector
  rx_cnt : Outport
  wires:
  Logical4/1 -> posedge1/1
  posedge1/1 -> payload_cnt2/2
  valid/1 -> Logical4/1
  eof/1 -> Logical4/2
  rst/1 -> payload_cnt2/1
  payload_cnt2/1 -> rx_cnt/1

== system b_r309c_med/Subsystem2 ==
  In1 : Inport  Port=1  LatchInput=off
  Constant7 : xbsIndex_r3/Constant  const=0  equ=P=C  arith_type=Unsigned  n_bits=16  bin_pt=0  opselect=C  inp2=PCIN>>17  opr=+  inp1=P  carry=CIN  iostate=0  explicit_period=on  period=1  dbl_ovrd=off
  Delay8 : xbsIndex_r3/Delay  latency=1  reg_retiming=on  explicit_period=off  period=1  en=off  accept_only_valid=off  init_zero=on  dbl_ovrd=off  show_param=off
      settings: xl_area=[0, 0, 0, 0, 0, 0, 0]
  Relational : xbsIndex_r3/Relational  mode=a!=b  latency=1  explicit_period=off  period=1  en=off  dbl_ovrd=off  show_param=off
      settings: xl_area=[0, 0, 0, 0, 0, 0, 0]
  Out1 : Outport
  wires:
  Delay8/1 -> Relational/1
  Constant7/1 -> Relational/2
  In1/1 -> Delay8/1
  Relational/1 -> Out1/1

== system b_r309c_med/Subsystem3 ==
  data_in : Inport  Port=1  LatchInput=off
  oob_in : Inport  Port=2  LatchInput=off
  we_in : Inport  Port=3  LatchInput=off
  link_down : Inport  Port=4  LatchInput=off
  Concat2 : xbsIndex_r3/Concat  num_inputs=2  explicit_period=off  period=1  dbl_ovrd=off
  Delay{1..2,4,6} (4 alike) : xbsIndex_r3/Delay  latency=2  reg_retiming=on  explicit_period=off  period=1  en=off  accept_only_valid=off  init_zero=on  dbl_ovrd=off  show_param=off
      settings: xl_area=[0, 0, 0, 0, 0, 0, 0]
  Slice9 : xbsIndex_r3/Slice  mode=Lower Bit Location + Width  nbits=1  bit1=0  base1=MSB of Input  bit0=1  base0=LSB of Input  boolean_output=on  explicit_period=off  period=1  dbl_ovrd=off
  data_out : Outport
  oob_out : Outport  Port=2
  trig_out : Outport  Port=3
  we_out : Outport  Port=4
  wires:
  Delay1/1 -> data_out/1
  Delay4/1 -> oob_out/1
  Delay6/1 -> trig_out/1
  oob_in/1 -> Slice9/1, Concat2/2
  Slice9/1 -> Delay6/1
  Delay2/1 -> we_out/1
  we_in/1 -> Delay2/1
  link_down/1 -> Concat2/1
  data_in/1 -> Delay1/1
  Concat2/1 -> Delay4/1

== system b_r309c_med/Subsystem4 ==
  rst : Inport  Port=1  LatchInput=off
  discard : Inport  Port=2  LatchInput=off
  eof : Inport  Port=3  LatchInput=off
  valid : Inport  Port=4  LatchInput=off
  Inverter3 : xbsIndex_r3/Inverter  latency=0  explicit_period=off  period=1  en=off  dbl_ovrd=off  show_param=off
      settings: xl_area=[0, 0, 0, 0, 0, 0, 0]
  Logical3 : xbsIndex_r3/Logical  logical_function=AND  inputs=3  precision=Full  arith_type=Unsigned  n_bits=8  bin_pt=2  align_bp=on  latency=0  explicit_period=on  period=1  en=off  dbl_ovrd=off  show_param=off
      settings: xl_area=[0, 0, 0, 0, 0, 0, 0]
  payload_cnt : xbsIndex_r3/Counter  cnt_type=Free Running  n_bits=32  bin_pt=0  arith_type=Unsigned  start_count=0  cnt_to=0  cnt_by_val=1  operation=Up  explicit_period=off  period=1  load_pin=off  rst=on  en=on  dbl_ovrd=off  show_param=off  use_rpm=on  gen_core=off
      settings: xl_area=[0, 0, 0, 0, 0, 0, 0]
  tx_cnt : Outport
  wires:
  Inverter3/1 -> Logical3/1
  Logical3/1 -> payload_cnt/2
  discard/1 -> Inverter3/1
  eof/1 -> Logical3/2
  valid/1 -> Logical3/3
  rst/1 -> payload_cnt/1
  payload_cnt/1 -> tx_cnt/1

== system b_r309c_med/Subsystem5 ==
  rst : Inport  Port=1  LatchInput=off
  we : Inport  Port=2  LatchInput=off
  eof : Inport  Port=3  LatchInput=off
  Logical2 : xbsIndex_r3/Logical  logical_function=AND  inputs=2  precision=Full  arith_type=Unsigned  n_bits=8  bin_pt=2  align_bp=on  latency=0  explicit_period=on  period=1  en=off  dbl_ovrd=off  show_param=off
      settings: xl_area=[0, 0, 0, 0, 0, 0, 0]
  payload_cnt1 : xbsIndex_r3/Counter  cnt_type=Free Running  n_bits=32  bin_pt=0  arith_type=Unsigned  start_count=0  cnt_to=0  cnt_by_val=1  operation=Up  explicit_period=on  period=1  load_pin=off  rst=on  en=on  dbl_ovrd=off  show_param=off  use_rpm=on  gen_core=off
      settings: xl_area=[0, 0, 0, 0, 0, 0, 0]
  posedge : casper_library/Misc/posedge  Tag=Rising Edge Detector
  rx_cnt : Outport
  wires:
  Logical2/1 -> posedge/1
  posedge/1 -> payload_cnt1/2
  we/1 -> Logical2/1
  eof/1 -> Logical2/2
  rst/1 -> payload_cnt1/1
  payload_cnt1/1 -> rx_cnt/1

== system b_r309c_med/Subsystem6 ==
  rst : Inport  Port=1  LatchInput=off
  discard : Inport  Port=2  LatchInput=off
  eof : Inport  Port=3  LatchInput=off
  valid : Inport  Port=4  LatchInput=off
  Inverter3 : xbsIndex_r3/Inverter  latency=0  explicit_period=off  period=1  en=off  dbl_ovrd=off  show_param=off
      settings: xl_area=[0, 0, 0, 0, 0, 0, 0]
  Logical3 : xbsIndex_r3/Logical  logical_function=AND  inputs=3  precision=Full  arith_type=Unsigned  n_bits=8  bin_pt=2  align_bp=on  latency=0  explicit_period=on  period=1  en=off  dbl_ovrd=off  show_param=off
      settings: xl_area=[0, 0, 0, 0, 0, 0, 0]
  payload_cnt : xbsIndex_r3/Counter  cnt_type=Free Running  n_bits=32  bin_pt=0  arith_type=Unsigned  start_count=0  cnt_to=0  cnt_by_val=1  operation=Up  explicit_period=off  period=1  load_pin=off  rst=on  en=on  dbl_ovrd=off  show_param=off  use_rpm=on  gen_core=off
      settings: xl_area=[0, 0, 0, 0, 0, 0, 0]
  tx_cnt : Outport
  wires:
  Inverter3/1 -> Logical3/1
  Logical3/1 -> payload_cnt/2
  discard/1 -> Inverter3/1
  eof/1 -> Logical3/2
  valid/1 -> Logical3/3
  rst/1 -> payload_cnt/1
  payload_cnt/1 -> tx_cnt/1

== system b_r309c_med/Subsystem7 ==
  data_in : Inport  Port=1  LatchInput=off
  valid_in : Inport  Port=2  LatchInput=off
  ip_in : Inport  Port=3  LatchInput=off
  eof_in : Inport  Port=4  LatchInput=off
  ibob_sync : Inport  Port=5  LatchInput=off
  xaui_down : Inport  Port=6  LatchInput=off
  ibob_mrst : Inport  Port=7  LatchInput=off
  ibob_pkt_err : Inport  Port=8  LatchInput=off
  Concat1 : xbsIndex_r3/Concat  num_inputs=6  explicit_period=off  period=1  dbl_ovrd=off
  Delay{1..4} (4 alike) : xbsIndex_r3/Delay  latency=2  reg_retiming=on  explicit_period=off  period=1  en=off  accept_only_valid=off  init_zero=on  dbl_ovrd=off  show_param=off
      settings: xl_area=[0, 0, 0, 0, 0, 0, 0]
  Logical4 : xbsIndex_r3/Logical  logical_function=AND  inputs=2  precision=Full  arith_type=Unsigned  n_bits=8  bin_pt=2  align_bp=on  latency=0  explicit_period=on  period=1  en=off  dbl_ovrd=off  show_param=off
      settings: xl_area=[0, 0, 0, 0, 0, 0, 0]
  Slice11 : xbsIndex_r3/Slice  mode=Lower Bit Location + Width  nbits=32-5  bit1=0  base1=MSB of Input  bit0=0  base0=LSB of Input  boolean_output=on  explicit_period=off  period=1  dbl_ovrd=off
  data_out : Outport
  oob_out : Outport  Port=2
  trig_out : Outport  Port=3
  we_out : Outport  Port=4
  wires:
  Slice11/1 -> Concat1/1
  Concat1/1 -> Delay4/1
  data_in/1 -> Delay1/1
  ip_in/1 -> Slice11/1
  Delay1/1 -> data_out/1
  Delay4/1 -> oob_out/1
  Logical4/1 -> Delay3/1
  valid_in/1 -> Logical4/2, Delay2/1
  eof_in/1 -> Concat1/2
  ibob_sync/1 -> Concat1/3, Logical4/1
  xaui_down/1 -> Concat1/4
  ibob_mrst/1 -> Concat1/5
  ibob_pkt_err/1 -> Concat1/6
  Delay2/1 -> we_out/1
  Delay3/1 -> trig_out/1

== system b_r309c_med/Subsystem8 ==
  In1 : Inport  Port=1  LatchInput=off
  In2 : Inport  Port=2  LatchInput=off
  Delay1 : xbsIndex_r3/Delay  latency=1  reg_retiming=on  explicit_period=off  period=1  en=off  accept_only_valid=off  init_zero=on  dbl_ovrd=off  show_param=off
      settings: xl_area=[0, 0, 0, 0, 0, 0, 0]
  Delay8 : xbsIndex_r3/Delay  latency=1  reg_retiming=on  explicit_period=off  period=1  en=off  accept_only_valid=off  init_zero=on  dbl_ovrd=off  show_param=off
      settings: xl_area=[0, 0, 0, 0, 0, 0, 0]
  Logical : xbsIndex_r3/Logical  logical_function=OR  inputs=2  precision=Full  arith_type=Unsigned  n_bits=8  bin_pt=2  align_bp=on  latency=0  explicit_period=off  period=1  en=off  dbl_ovrd=off  show_param=off
      settings: xl_area=[0, 0, 0, 0, 0, 0, 0]
  pulse_ext : Subsystem  mask{pulse_len=2^23}
      mask prompts: pulse_len "Length of Pulse"
      mask init:
      | bits = ceil(log2(pulse_len));
  Out1 : Outport
  wires:
  In1/1 -> Delay8/1
  pulse_ext/1(out) -> Out1/1
  Logical/1 -> pulse_ext/1(in)
  In2/1 -> Delay1/1
  Delay8/1 -> Logical/1
  Delay1/1 -> Logical/2

== system b_r309c_med/Subsystem9 ==
  data_in : Inport  Port=1  LatchInput=off
  oob_in : Inport  Port=2  LatchInput=off
  we_in : Inport  Port=3  LatchInput=off
  link_down : Inport  Port=4  LatchInput=off
  Concat2 : xbsIndex_r3/Concat  num_inputs=2  explicit_period=off  period=1  dbl_ovrd=off
  Delay{1..2,4,6} (4 alike) : xbsIndex_r3/Delay  latency=2  reg_retiming=on  explicit_period=off  period=1  en=off  accept_only_valid=off  init_zero=on  dbl_ovrd=off  show_param=off
      settings: xl_area=[0, 0, 0, 0, 0, 0, 0]
  Slice9 : xbsIndex_r3/Slice  mode=Lower Bit Location + Width  nbits=1  bit1=0  base1=MSB of Input  bit0=1  base0=LSB of Input  boolean_output=on  explicit_period=off  period=1  dbl_ovrd=off
  data_out : Outport
  oob_out : Outport  Port=2
  trig_out : Outport  Port=3
  we_out : Outport  Port=4
  wires:
  Delay1/1 -> data_out/1
  Delay4/1 -> oob_out/1
  Delay6/1 -> trig_out/1
  oob_in/1 -> Slice9/1, Concat2/2
  Slice9/1 -> Delay6/1
  Delay2/1 -> we_out/1
  we_in/1 -> Delay2/1
  link_down/1 -> Concat2/1
  data_in/1 -> Delay1/1
  Concat2/1 -> Delay4/1
